simulink model "Simulation_PIL"  (R2023b)
settings: Solver=FixedStepAuto  StartTime=0.0  StopTime=2  RelTol=1e-3  EnableMultiTasking=on
undefined symbols (not defined in the file or in its folder): bldc, inverter, PI_params, PWM_frequency, target, Ts, Ts_motor, Ts_motor_simscape, Ts_simulink, Ts_speed
libraries: nesl_utility x26, fl_lib x16, ee_lib x10, mcbcontrolslib x8, simulink x6, mcbpositiondecoderlib x5, slpidlib x4, pil_lib x1
(part 3 of 3)

== system Simulation_PIL/Inverter and Motor2/Sensor_Measurements/Halls/Hall State Plant to HW/If Action Subsystem5 ==
  Action Port : ActionPort  ActionPortLabel=case [ 3 ]:
  Constant : Constant  Value=bldc.HallSequence(6)  OutDataTypeStr=uint16
  Out1 : Outport
  wires:
  Constant/1 -> Out1/1

== system Simulation_PIL/Inverter and Motor2/Inverter and Motor/Subsystem1/Sensing w a/Hall sensor/Subsystem ==
  theta : Inport
  Trigonometric Function : Trigonometry  Operator=sincos
  Trigonometric Function2 : Trigonometry  Operator=atan2
  mech->elec : Gain  Gain=bldc.p
  rad->deg : Gain  Gain=180/pi  SaturateOnIntegerOverflow=on  OutDataTypeStr=Inherit: Same as input  ParamDataTypeStr=Inherit: Same as input
  deg : Outport  VectorParamsAs1DForOutWhenUnconnected=off
  wires:
  mech->elec/1 -> Trigonometric Function/1
  Trigonometric Function/2 -> Trigonometric Function2/2
  rad->deg/1 -> deg/1
  theta/1 -> mech->elec/1
  Trigonometric Function/1 -> Trigonometric Function2/1
  Trigonometric Function2/1 -> rad->deg/1
